simulink model "PI_only_theta"  (R2021a)
settings: Solver=VariableStepAuto  StartTime=0.0  StopTime=10.0  RelTol=1e-3
values from neighbouring files (symbols this model uses):
  dem = syscomp_JC.Denominator{:}    [Compensator_schemes.m]    (also in PI_Controller_script.m = syscomp.Denominator{:}; PI_Ziegler-Nichols (not good).m = syscomp.Denominator{:}; PI_controller.m = syscomp.Denominator{:})
  Gp = tf(sysestc)    [rlocusPI.m]
  Kp = Kp *0.5    [PI_Controller_script.m]    (also in PI_Ziegler-Nichols (not good).m; PI_controller.m = 0.9*Tpid/(Kpid*Lpid); rlocusPI.m = 2.6464)
  num = syscomp_JC.Numerator{:}    [Compensator_schemes.m]    (also in PI_Controller_script.m = syscomp.Numerator{:}; PI_Ziegler-Nichols (not good).m = syscomp.Numerator{:}; PI_controller.m = syscomp.Numerator{:}; rlocusPI.m = Gp(1).Numerator{:})
  Ti = Ti * 20000    [PI_Controller_script.m]    (also in PI_Ziegler-Nichols (not good).m; PI_controller.m = 3*Lpid; rlocusPI.m = 1.1)
undefined symbols (not defined in the file or in its folder): sigbuilder_block
libraries: cstblocks x1
settings Model: Creator=jesuc  LastModifiedBy=arco

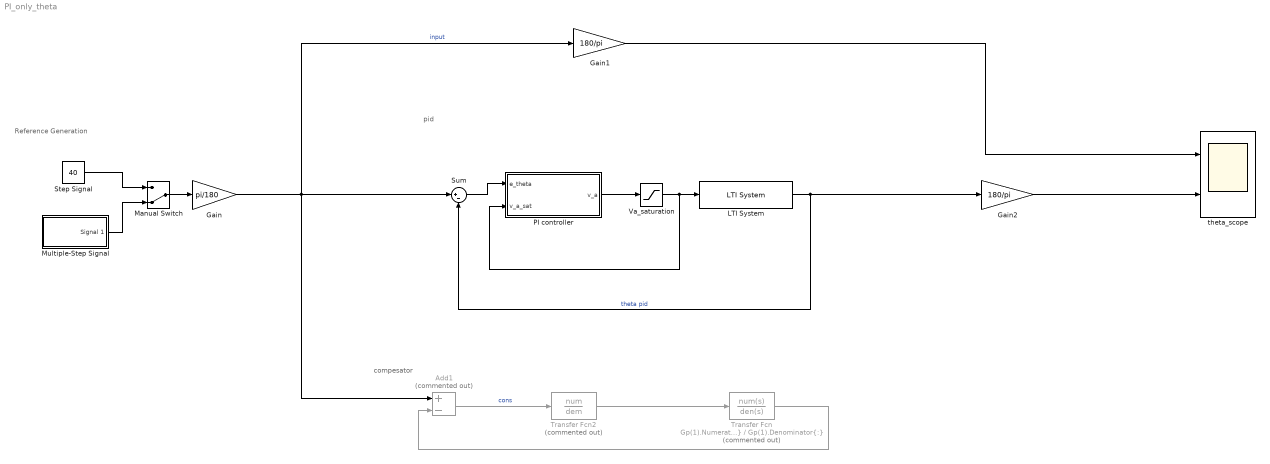
== system PI_only_theta ==
  note: pid
  note: compesator
  note: Reference Generation
  Add1 : Sum  Commented=on  Inputs=+-
  Gain : Gain  Gain=pi/180
  Gain1 : Gain  Gain=180/pi
  Gain2 : Gain  Gain=180/pi
  LTI System : cstblocks/LTI System  sys=G_theta_cont  IC=[]
  Manual Switch : ManualSwitch  CurrentSetting=0
  Multiple-Step Signal : Subsystem  Tag=STV Subsys  LoadFcn=sigbuilder_block('load');  StartFcn=sigbuilder_block('start');  StopFcn=sigbuilder_block('stop');  ClipboardFcn=sigbuilder_block('clipboard');  mask(Sigbuilder block){tuvar=[0:10]}
      mask help: Simulink:masks:SigbuilderBlock_MD
      mask init:
      | if ~strcmp(get_param(bdroot(gcbh),'SimulationStatus'),'stopped') tuvar = sigbuilder_block('maskInit'); end
      settings: CopyFcn=sigbuilder_block('copy');  DeleteFcn=sigbuilder_block('delete');  ModelCloseFcn=sigbuilder_block('modelClose');  PreSaveFcn=sigbuilder_block('preSave');  PauseFcn=sigbuilder_block('pause');  ContinueFcn=sigbuilder_block('continue');  NameChangeFcn=sigbuilder_block('namechange');  OpenFcn=sigbuilder_block('open',[437.6 199.2 550.4 400 ]);  CloseFcn=sigbuilder_block('close');
      mask Display: plot(0, 0, 100, 100,[2, 2, 32, 32, 2], [68, 8, 8, 68, 68],[32, 2], [38, 38], [32, 19, 2],[53, 60, 44], [32, 17, 17, 2],[16, 16, 31, 31]);txt = getActiveGroup(gcbh);text(2, 100, txt,'verticalAlignment', 'top');
  PI controller : Subsystem
  Step Signal : Constant  Value=40
  Sum : Sum  Inputs=|+-
  Transfer Fcn : TransferFcn  Commented=on  Numerator=Gp(1).Numerator{:}  Denominator=Gp(1).Denominator{:}
  Transfer Fcn2 : TransferFcn  Commented=on  Numerator=num  Denominator=dem
  Va_saturation : Saturate  UpperLimit=5  LowerLimit=-5
  theta_scope : Scope  NumInputPorts=2
  wires:
  LTI System/1 -> Gain2/1, Sum/2  "theta pid"
  Transfer Fcn2/1 -> Transfer Fcn/1
  Transfer Fcn/1 -> Add1/2
  Add1/1 -> Transfer Fcn2/1  "cons"
  Va_saturation/1 -> PI controller/2(v_a_sat), LTI System/1
  Gain/1 -> Add1/1, Sum/1, Gain1/1  "input"
  Multiple-Step Signal/1(Signal 1) -> Manual Switch/2
  Step Signal/1 -> Manual Switch/1
  Manual Switch/1 -> Gain/1
  Gain1/1 -> theta_scope/1
  Sum/1 -> PI controller/1(e_theta)
  PI controller/1(v_a) -> Va_saturation/1
  Gain2/1 -> theta_scope/2

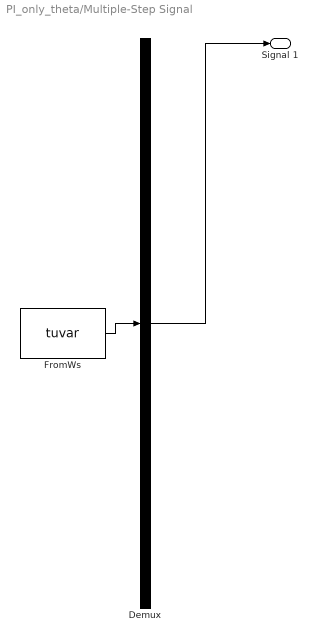
== system PI_only_theta/Multiple-Step Signal ==
  Demux : Demux  Tag=STV Demux  Outputs=1
      settings: DisplayOption=none
  FromWs : FromWorkspace  Tag=STV FromWs  VariableName=tuvar
      SigBuilderData=|
      | common.afterFinalStr = 'Extrapolate'
      | common.sampleTime = 0
      | dataSet.timeRange = [0 10]
      | dataSet.name = 'Group 1'
      | sbobj.Groups.Name = 'Group 1'
      | sbobj.Groups.Signals.Name = 'Signal 1'
      | sbobj.Groups.Signals.XData = [0 1 1 3 3 5 5 7 7 8.5 8.5 10]
      | sbobj.Groups.Signals.YData = [0.005 0.005 40 40 15 15 -30 -30 0 0 23 23]
  Signal 1 : Outport  Tag=STV Outport
  wires:
  Demux/1 -> Signal 1/1
  FromWs/1 -> Demux/1

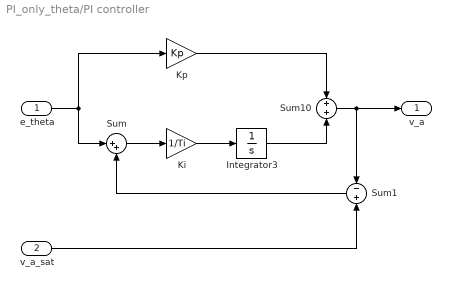
== system PI_only_theta/PI controller ==
  e_theta : Inport
  v_a_sat : Inport  Port=2
  Integrator3 : Integrator
  Ki : Gain  Gain=1/Ti
  Kp : Gain  Gain=Kp
  Sum : Sum  Inputs=|++
  Sum1 : Sum  Inputs=-+
  Sum10 : Sum
  v_a : Outport
  wires:
  e_theta/1 -> Sum/1, Kp/1
  Ki/1 -> Integrator3/1
  Sum10/1 -> v_a/1, Sum1/1
  Integrator3/1 -> Sum10/2
  Kp/1 -> Sum10/1
  Sum/1 -> Ki/1
  v_a_sat/1 -> Sum1/2
  Sum1/1 -> Sum/2
